simulink library "neuromorphic_blocks"  (R2022a)
settings: Solver=VariableStepAuto  StartTime=0.0  StopTime=10.0  RelTol=1e-3
libraries: $bdroot x31, simulink x7
(part 2 of 2)

== system neuromorphic_blocks/Secondary Blocks ==
  Event Demux : Subsystem  mask(Event Demux){symmetric_box=off, dsyn_signal_pos=0, dsyn_signal_neg=0, dsyn_signal_neg_save=0, gain_signal_pos=1, gain_signal_neg=1, gain_signal_neg_save=1, input=Events, gsyn_pos=0, gsyn_neg=0, gsyn_neg_save=0, dsyn_event_pos=0, dsyn_event_neg=0, dsyn_event_neg_save=0, gain_event_pos=1, gain_event_neg=1, gain_event_neg_save=1}
      mask prompts: symmetric_box "Differentiate positive and negative parameters"; dsyn_signal_pos "Value"; dsyn_signal_neg "Neg"; dsyn_signal_neg_save "Save"; gain_signal_pos "Value"; gain_signal_neg "Neg"; gain_signal_neg_save "Save"; gsyn_pos "Value"; gsyn_neg "Neg"; gsyn_neg_save "Save"; dsyn_event_pos "Value"; dsyn_event_neg "Neg"; dsyn_event_neg_save "Save"; gain_event_pos "Value"; gain_event_neg "Neg"; gain_event_neg_save "Save"
      mask init:
      | mask  = Simulink.Mask.get(gcb);
      |     switch mask.getParameter('input').Value
      |         case 'Events'
      |             %set_param([gcb '/VSNK_ev' ],'LabelModeActiveChoice', 'Events');
      |             %set_param([gcb '/VSNK_s' ],'LabelModeActiveChoice', 'Events');
      |             %set_param([gcb '/VSRC' ],'LabelModeActiveChoice', 'Events');
      |             set_param([gcb '/VSub' ],'LabelModeActiveChoice', 'Events');
      |             %mask.getPortConstraint('inout_main_type').Rule.DataType = {'boolean'};
      |             try
      |                 set_param([gcb '/V'], 'Name', 'Ev');
      |                 set_param([gcb '/V+'], 'Name', 'Ev+');
      |                 set_param([gcb '/V-'], 'Name', 'Ev-');
      |             catch E
      |             end
      |         case 'Voltage'
      |             %set_param([gcb '/VSNK_ev' ],'LabelModeActiveChoice', 'Voltage');
      |             %set_param([gcb '/VSNK_s' ],'LabelModeActiveChoice', 'Voltage');
      |             %set_param([gcb '/VSRC' ],'LabelModeActiveChoice', 'Voltage');
      |             set_param([gcb '/VSub' ],'LabelModeActiveChoice', 'Voltage');
      |             %mask.getPortConstraint('inout_main_type').Rule.DataType = {'double'; 'single'; 'int8'; 'uint8'; 'int16'; 'uint16'; 'int32'; 'uint32'};
      |             try
      |                 set_param([gcb '/Ev'], 'Name', 'V');
      |                 set_param([gcb '/Ev+'], 'Name', 'V+');
      |                 set_param([gcb '/Ev-'], 'Name', 'V-');
      |             catch E
      |             end
      |     end
      | 
      |     suffix_list = {'gsyn', 'dsyn_event', 'gain_event', 'dsyn_signal', 'gain_signal'};
      |     switch mask.getParameter('symmetric_box').Value
      |         case 'off'
      |             for suffix_cell = suffix_list
      |                 suffix = suffix_cell{1};
      |                 mask.getParameter([suffix '_neg']).Value = mask.getParameter([suffix '_pos']).Value;
      |             end
      |         case 'on'
      |             for suffix_cell = suffix_list
      |                 suffix = suffix_cell{1};
      |                 mask.getParameter([suffix '_neg']).Value = mask.getParameter([suffix '_neg_save']).Value;
      |             end
      |     end
      mask Callback symmetric_box:
      | mask  = Simulink.Mask.get(gcb);
      |     switch mask.getParameter('input').Value
      |         case 'Events'
      |             suffix_list = {'dsyn_signal', 'gain_signal'};
      |         case 'Voltage'
      |             suffix_list = {'dsyn_signal', 'gain_signal', 'gsyn', 'dsyn_event', 'gain_event'};
      |     end
      | 
      |     switch mask.getParameter('symmetric_box').Value
      |         case 'on'
      |             for suffix_cell = suffix_list
      |                 suffix = suffix_cell{1};
      |                 %mask.getParameter([suffix '_neg']).Hidden = 'off';
      |                 %mask.getParameter([suffix '_neg_save']).ReadOnly = 'off';
      |                 mask.getParameter([suffix '_neg']).Value = mask.getParameter([suffix '_neg_save']).Value;
      |                 %mask.getParameter([suffix '_neg']).Enabled = 'on';
      |                 mask.getParameter([suffix '_neg']).Visible = 'on';
      |                 mask.getParameter([suffix '_pos']).Prompt = 'Pos';
      |             end
      |         case 'off'
      |             for suffix_cell = suffix_list
      |                 suffix = suffix_cell{1};
      |                 %mask.getParameter([suffix '_neg_save']).Value = mask.getParameter([suffix '_neg']).Value;
      |                 %mask.getParameter([suffix '_neg_save']).ReadOnly = 'on';
      |                 %mask.getParameter([suffix '_neg']).Enabled = 'off';
      |                 mask.getParameter([suffix '_neg']).Visible = 'off';
      |                 mask.getParameter([suffix '_pos']).Prompt = 'Value';
      |                 %mask.getParameter([suffix '_neg']).Value = mask.getParameter([suffix '_pos']).Value;
      |                 %mask.getParameter([suffix '_neg']).Hidden = 'on';
      |             end
      |     end
      mask Callback dsyn_signal_neg:
      | suffix = 'dsyn_signal';
      |     mask  = Simulink.Mask.get(gcb);
      |     switch mask.getParameter('symmetric_box').Value
      |         case 'on'
      |              mask.getParameter([suffix '_neg_save']).Value = mask.getParameter([suffix '_neg']).Value;
      |     end
      mask Callback gain_signal_neg:
      | suffix = 'gain_signal';
      |     mask  = Simulink.Mask.get(gcb);
      |     switch mask.getParameter('symmetric_box').Value
      |         case 'on'
      |              mask.getParameter([suffix '_neg_save']).Value = mask.getParameter([suffix '_neg']).Value;
      |     end
      mask TypeOptions input: Events | Voltage
      mask Callback input:
      | mask = Simulink.Mask.get(gcb);
      |     suffix_list = {'gsyn', 'dsyn_event', 'gain_event'};
      |     switch mask.getParameter('input').Value
      |         case 'Events'
      |             for suffix_cell = suffix_list
      |                 suffix = suffix_cell{1};
      |                 %mask.getParameter([suffix '_pos']).Enabled = 'off';
      |                 mask.getParameter([suffix '_pos']).Visible = 'off';
      |                 %mask.getParameter([suffix '_neg']).Enabled = 'off';
      |                 mask.getParameter([suffix '_neg']).Visible = 'off';
      |                 %mask.getDialogControl([suffix '_text']).Enabled = 'off';
      |                 mask.getDialogControl([suffix '_text']).Visible = 'off';
      |             end
      |         case 'Voltage'
      |             switch mask.getParameter('symmetric_box').Value
      |                 case 'on'
      |                     enable_neg = true;
      |                 case 'off'
      |                     enable_neg = false;
      |             end
      |             for suffix_cell = suffix_list
      |                 suffix = suffix_cell{1};
      |                 %mask.getParameter([suffix '_pos']).Enabled = 'on';
      |                 mask.getParameter([suffix '_pos']).Visible = 'on';
      |                 %mask.getDialogControl([suffix '_text']).Enabled = 'on';
      |                 mask.getDialogControl([suffix '_text']).Visible = 'on';
      |                 if enable_neg
      |                     %mask.getParameter([suffix '_neg']).Enabled = 'on';
      |                     mask.getParameter([suffix '_neg']).Visible = 'on';
      |                 end
      |             end
      |     end
      mask Callback gsyn_neg:
      | suffix = 'gsyn';
      |     mask  = Simulink.Mask.get(gcb);
      |     switch mask.getParameter('symmetric_box').Value
      |         case 'on'
      |              mask.getParameter([suffix '_neg_save']).Value = mask.getParameter([suffix '_neg']).Value;
      |     end
      mask Callback dsyn_event_neg:
      | suffix = 'dsyn_event';
      |     mask  = Simulink.Mask.get(gcb);
      |     switch mask.getParameter('symmetric_box').Value
      |         case 'on'
      |              mask.getParameter([suffix '_neg_save']).Value = mask.getParameter([suffix '_neg']).Value;
      |     end
      mask Callback gain_event_neg:
      | suffix = 'gain_event';
      |     mask  = Simulink.Mask.get(gcb);
      |     switch mask.getParameter('symmetric_box').Value
      |         case 'on'
      |              mask.getParameter([suffix '_neg_save']).Value = mask.getParameter([suffix '_neg']).Value;
      |     end
      mask DialogControl dsyn_signal_text Prompt: Signal Bias
      mask DialogControl gain_signal_text Prompt: Signal Slope
      mask DialogControl input_text Prompt: Input-Output Type
      mask DialogControl gsyn_text Prompt: Event Gain
      mask DialogControl dsyn_event_text Prompt: Event Bias
      mask DialogControl gain_event_text Prompt: Event Slope
      mask Display:
      | simBlockH = get_param(gcb, 'Handle');
      | 
      | 
      | portH = find_system(simBlockH, 'LookUnderMasks', 'on', 'FollowLinks', 'on', 'SearchDepth', 1, 'BlockType', 'Inport');
      | portNames = cellstr(get_param(portH, 'Name'));
      | portNum = cellstr(get_param(portH, 'Port'));
      | for i = 1:length(portNames)
      |     if ~isempty(portNames{i})
      |         num = str2num(['uint8(' portNum{i} ')']);
      |         port_label('input', num, portNames{i});
      |     end
      | end
      | 
      | portH = find_system(simBlockH, 'LookUnderMasks', 'on', 'FollowLinks', 'on', 'SearchDepth', 1, 'BlockType', 'Outport');
      | portNames = cellstr(get_param(portH, 'Name'));
      | portNum = cellstr(get_param(portH, 'Port'));
      | for i = 1:length(portNames)
      |     if ~isempty(portNames{i})
      |         num = str2num(['uint8(' portNum{i} ')']);
      |         port_label('output', num, portNames{i});
      |     end
      | end
  Event Mux : Subsystem  mask(Event Mux){symmetric_box=off, dsyn_signal_pos=0, dsyn_signal_neg=0, dsyn_signal_neg_save=0, gain_signal_pos=1, gain_signal_neg=1, gain_signal_neg_save=1, input=Events, gsyn_pos=0, gsyn_neg=0, gsyn_neg_save=0, dsyn_event_pos=0, dsyn_event_neg=0, dsyn_event_neg_save=0, gain_event_pos=1, gain_event_neg=1, gain_event_neg_save=1}
      mask prompts: symmetric_box "Differentiate positive and negative parameters"; dsyn_signal_pos "Value"; dsyn_signal_neg "Neg"; dsyn_signal_neg_save "Save"; gain_signal_pos "Value"; gain_signal_neg "Neg"; gain_signal_neg_save "Save"; gsyn_pos "Value"; gsyn_neg "Neg"; gsyn_neg_save "Save"; dsyn_event_pos "Value"; dsyn_event_neg "Neg"; dsyn_event_neg_save "Save"; gain_event_pos "Value"; gain_event_neg "Neg"; gain_event_neg_save "Save"
      mask init: same as neuromorphic_blocks/Secondary Blocks/Event Demux
      mask Callback symmetric_box:
      | mask  = Simulink.Mask.get(gcb);
      |     switch mask.getParameter('input').Value
      |         case 'Events'
      |             suffix_list = {'dsyn_signal', 'gain_signal'};
      |         case 'Voltage'
      |             suffix_list = {'dsyn_signal', 'gain_signal', 'gsyn', 'dsyn_event', 'gain_event'};
      |     end
      | 
      |     switch mask.getParameter('symmetric_box').Value
      |         case 'on'
      |             for suffix_cell = suffix_list
      |                 suffix = suffix_cell{1};
      |                 %mask.getParameter([suffix '_neg']).Hidden = 'off';
      |                 %mask.getParameter([suffix '_neg_save']).ReadOnly = 'off';
      |                 mask.getParameter([suffix '_neg']).Value = mask.getParameter([suffix '_neg_save']).Value;
      |                 %mask.getParameter([suffix '_neg']).Enabled = 'on';
      |                 mask.getParameter([suffix '_neg']).Visible = 'on';
      |                 mask.getParameter([suffix '_pos']).Prompt = 'Pos';
      |             end
      |         case 'off'
      |             for suffix_cell = suffix_list
      |                 suffix = suffix_cell{1};
      |                 %mask.getParameter([suffix '_neg_save']).Value = mask.getParameter([suffix '_neg']).Value;
      |                 %mask.getParameter([suffix '_neg_save']).ReadOnly = 'on';
      |                 %mask.getParameter([suffix '_neg']).Enabled = 'off';
      |                 mask.getParameter([suffix '_neg']).Visible = 'off';
      |                 mask.getParameter([suffix '_pos']).Prompt = 'Value';
      |                 %mask.getParameter([suffix '_neg']).Value = mask.getParameter([suffix '_pos']).Value;
      |                 %mask.getParameter([suffix '_neg']).Hidden = 'on';
      |             end
      |     end
      mask Callback dsyn_signal_neg:
      | suffix = 'dsyn_signal';
      |     mask  = Simulink.Mask.get(gcb);
      |     switch mask.getParameter('symmetric_box').Value
      |         case 'on'
      |              mask.getParameter([suffix '_neg_save']).Value = mask.getParameter([suffix '_neg']).Value;
      |     end
      mask Callback gain_signal_neg:
      | suffix = 'gain_signal';
      |     mask  = Simulink.Mask.get(gcb);
      |     switch mask.getParameter('symmetric_box').Value
      |         case 'on'
      |              mask.getParameter([suffix '_neg_save']).Value = mask.getParameter([suffix '_neg']).Value;
      |     end
      mask TypeOptions input: Events | Voltage
      mask Callback input:
      | mask = Simulink.Mask.get(gcb);
      |     suffix_list = {'gsyn', 'dsyn_event', 'gain_event'};
      |     switch mask.getParameter('input').Value
      |         case 'Events'
      |             for suffix_cell = suffix_list
      |                 suffix = suffix_cell{1};
      |                 %mask.getParameter([suffix '_pos']).Enabled = 'off';
      |                 mask.getParameter([suffix '_pos']).Visible = 'off';
      |                 %mask.getParameter([suffix '_neg']).Enabled = 'off';
      |                 mask.getParameter([suffix '_neg']).Visible = 'off';
      |                 %mask.getDialogControl([suffix '_text']).Enabled = 'off';
      |                 mask.getDialogControl([suffix '_text']).Visible = 'off';
      |             end
      |         case 'Voltage'
      |             switch mask.getParameter('symmetric_box').Value
      |                 case 'on'
      |                     enable_neg = true;
      |                 case 'off'
      |                     enable_neg = false;
      |             end
      |             for suffix_cell = suffix_list
      |                 suffix = suffix_cell{1};
      |                 %mask.getParameter([suffix '_pos']).Enabled = 'on';
      |                 mask.getParameter([suffix '_pos']).Visible = 'on';
      |                 %mask.getDialogControl([suffix '_text']).Enabled = 'on';
      |                 mask.getDialogControl([suffix '_text']).Visible = 'on';
      |                 if enable_neg
      |                     %mask.getParameter([suffix '_neg']).Enabled = 'on';
      |                     mask.getParameter([suffix '_neg']).Visible = 'on';
      |                 end
      |             end
      |     end
      mask Callback gsyn_neg:
      | suffix = 'gsyn';
      |     mask  = Simulink.Mask.get(gcb);
      |     switch mask.getParameter('symmetric_box').Value
      |         case 'on'
      |              mask.getParameter([suffix '_neg_save']).Value = mask.getParameter([suffix '_neg']).Value;
      |     end
      mask Callback dsyn_event_neg:
      | suffix = 'dsyn_event';
      |     mask  = Simulink.Mask.get(gcb);
      |     switch mask.getParameter('symmetric_box').Value
      |         case 'on'
      |              mask.getParameter([suffix '_neg_save']).Value = mask.getParameter([suffix '_neg']).Value;
      |     end
      mask Callback gain_event_neg:
      | suffix = 'gain_event';
      |     mask  = Simulink.Mask.get(gcb);
      |     switch mask.getParameter('symmetric_box').Value
      |         case 'on'
      |              mask.getParameter([suffix '_neg_save']).Value = mask.getParameter([suffix '_neg']).Value;
      |     end
      mask DialogControl dsyn_signal_text Prompt: Signal Bias
      mask DialogControl gain_signal_text Prompt: Signal Slope
      mask DialogControl input_text Prompt: Input-Output Type
      mask DialogControl gsyn_text Prompt: Event Gain
      mask DialogControl dsyn_event_text Prompt: Event Bias
      mask DialogControl gain_event_text Prompt: Event Slope
      mask Display:
      | simBlockH = get_param(gcb, 'Handle');
      | 
      | 
      | portH = find_system(simBlockH, 'LookUnderMasks', 'on', 'FollowLinks', 'on', 'SearchDepth', 1, 'BlockType', 'Inport');
      | portNames = cellstr(get_param(portH, 'Name'));
      | portNum = cellstr(get_param(portH, 'Port'));
      | for i = 1:length(portNames)
      |     if ~isempty(portNames{i})
      |         num = str2num(['uint8(' portNum{i} ')']);
      |         port_label('input', num, portNames{i});
      |     end
      | end
      | 
      | portH = find_system(simBlockH, 'LookUnderMasks', 'on', 'FollowLinks', 'on', 'SearchDepth', 1, 'BlockType', 'Outport');
      | portNames = cellstr(get_param(portH, 'Name'));
      | portNum = cellstr(get_param(portH, 'Port'));
      | for i = 1:length(portNames)
      |     if ~isempty(portNames{i})
      |         num = str2num(['uint8(' portNum{i} ')']);
      |         port_label('output', num, portNames{i});
      |     end
      | end
  Noise on Signal : Subsystem  mask(Noise on Signal){noise_pwr=0, timescale=0.004, rel_timescale=1, seed=-1, seed_mem=randi([0, 100000])}
      mask prompts: noise_pwr "Value"; timescale "Value"; rel_timescale "Value"; seed "Value"
      mask init: same as neuromorphic_blocks/Events Transmission Blocks/Event Loss
      mask DialogControl noise_pwr_text Prompt: Noise Power
      mask DialogControl timescale_text Prompt: Timescale
      mask DialogControl rel_timescale_text Prompt: Relative Timescale
      mask DialogControl seed_text Prompt: Seed (-1 for random seed)
      mask Display:
      | xscale = 0.8;
      | yscale = 0.8;
      | 
      | r = [-0.4326
      |    -1.6656
      |     0.1253
      |     0.2877
      |    -1.1465
      |     1.1909
      |     1.1892
      |    -0.0376
      |     0.3273
      |     0.1746
      |    -0.1867
      |     0.7258]';
      | 
      | r2 = repelem(r,2);
      | r3 = r2 - min(r2);
      | r4 = r3/max(r3);
      | r5 = r4*yscale + (1-yscale)/2;
      | 
      | 
      | t = [1 repelem(2:12,2) 13];
      | t2 = t - min(t);
      | t3 = t2/max(t2);
      | t4 = t3*xscale + (1-xscale)/2;
      | 
      | 
      | plot(t4, r5);

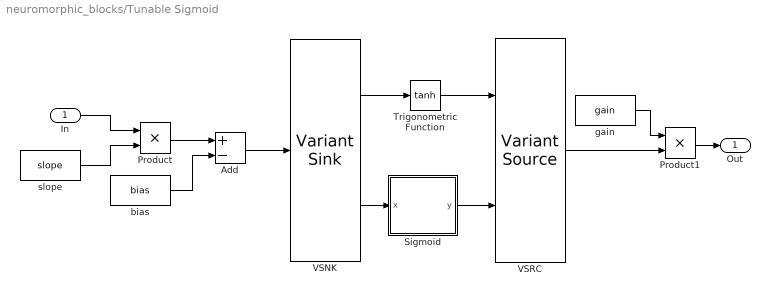
== system neuromorphic_blocks/Tunable Sigmoid ==
  In : Inport
  Add : Sum  Inputs=+-
  Product : Product
  Product1 : Product
  Sigmoid : Subsystem
  Trigonometric Function : Trigonometry  Operator=tanh
  VSNK : VariantSink  VariantControlMode=label  LabelModeActiveChoice=Sigmoid  ShowConditionOnBlock=on
  VSRC : VariantSource  VariantControlMode=label  LabelModeActiveChoice=Sigmoid  ShowConditionOnBlock=on
  bias : Constant  Value=bias
  gain : Constant  Value=gain
  slope : Constant  Value=slope
  Out : Outport
  wires:
  VSNK/1 -> Trigonometric Function/1
  slope/1 -> Product/2
  In/1 -> Product/1
  Add/1 -> VSNK/1
  Product/1 -> Add/1
  bias/1 -> Add/2
  VSRC/1 -> Product1/2
  Product1/1 -> Out/1
  gain/1 -> Product1/1
  VSNK/2 -> Sigmoid/1(x)
  Sigmoid/1(y) -> VSRC/2
  Trigonometric Function/1 -> VSRC/1

== system neuromorphic_blocks/Events Transmission Blocks/Continuous to Event ==
  In : Inport
  Constant2 : Constant  Value=thresh
  Relational Operator : RelationalOperator  OutDataTypeStr=boolean  RndMeth=Simplest  InputSameDT=off
  Out : Outport  OutDataTypeStr=boolean
  wires:
  Constant2/1 -> Relational Operator/2
  In/1 -> Relational Operator/1
  Relational Operator/1 -> Out/1

== system neuromorphic_blocks/Events Transmission Blocks/Event Loss ==
  In : Inport
  Constant4 : Constant  Value=0  OutDataTypeStr=Inherit: Inherit via back propagation
  Generate Random Number on Positive : Subsystem  TreatAsAtomicUnit=on
  Pipe Signal : Switch  Threshold=loss_prob  SaturateOnIntegerOverflow=off  InputSameDT=off
  Out : Outport
  wires:
  Generate Random Number on Positive/1(Out1) -> Pipe Signal/2
  In/1 -> Pipe Signal/1, Generate Random Number on Positive/Trigger
  Constant4/1 -> Pipe Signal/3
  Pipe Signal/1 -> Out/1

== system neuromorphic_blocks/Events Transmission Blocks/Event to Continuous ==
  In : Inport  OutDataTypeStr=boolean
  Gain : Gain  Gain=gain  OutDataTypeStr=double
  Out : Outport  OutDataTypeStr=double
  wires:
  In/1 -> Gain/1
  Gain/1 -> Out/1

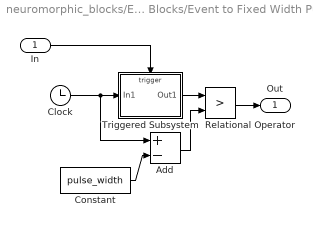
== system neuromorphic_blocks/Events Transmission Blocks/Event to Fixed Width Pulse ==
  In : Inport
  Add : Sum  Inputs=+-
  Clock : Clock
  Constant : Constant  Value=pulse_width
  Relational Operator : RelationalOperator  Operator=>  OutDataTypeStr=boolean  RndMeth=Simplest  InputSameDT=off
  Triggered Subsystem : Subsystem  TreatAsAtomicUnit=on
  Out : Outport
  wires:
  Constant/1 -> Add/2
  Triggered Subsystem/1(Out1) -> Relational Operator/1
  Add/1 -> Relational Operator/2
  Clock/1 -> Add/1, Triggered Subsystem/1(In1)
  Relational Operator/1 -> Out/1
  In/1 -> Triggered Subsystem/Trigger

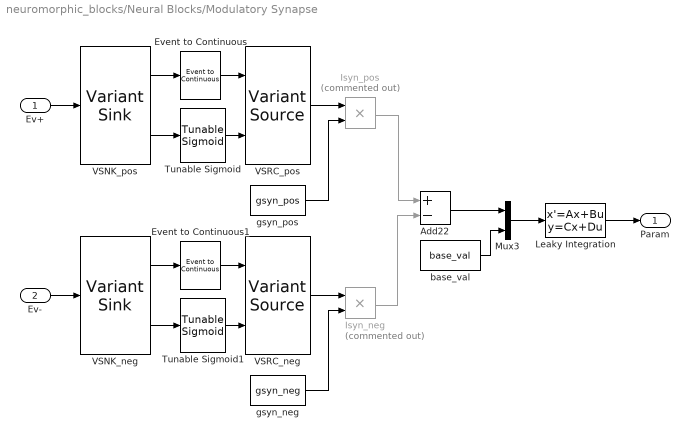
== system neuromorphic_blocks/Neural Blocks/Modulatory Synapse ==
  Ev+ : Inport
  Ev- : Inport  Port=2
  Add22 : Sum  Inputs=+-
  Event to Continuous : $bdroot/Events Transmission Blocks/Event to Continuous  gain=1
  Event to Continuous1 : $bdroot/Events Transmission Blocks/Event to Continuous  gain=1
  Isyn_neg : Product  Commented=on
  Isyn_pos : Product  Commented=on
  Leaky Integration : StateSpace  A=-1/(timescale*rel_timescale)  B=[1 1/(timescale*rel_timescale)]  D=[0 0]  InitialCondition=base_val  ParameterTunability=Unconstrained
  Mux3 : Mux  Inputs=2
  Tunable Sigmoid : $bdroot/Tunable Sigmoid  nonlinearity_type=Sigmoid  gain_source=Internal  gain=1  bias=dsyn_pos  slope=msyn_pos
  Tunable Sigmoid1 : $bdroot/Tunable Sigmoid  nonlinearity_type=Sigmoid  gain_source=Internal  gain=1  bias=dsyn_neg  slope=msyn_neg
  VSNK_neg : VariantSink  VariantControlMode=label  LabelModeActiveChoice=Events  ShowConditionOnBlock=on
  VSNK_pos : VariantSink  VariantControlMode=label  LabelModeActiveChoice=Events  ShowConditionOnBlock=on
  VSRC_neg : VariantSource  VariantControlMode=label  LabelModeActiveChoice=Events  ShowConditionOnBlock=on
  VSRC_pos : VariantSource  VariantControlMode=label  LabelModeActiveChoice=Events  ShowConditionOnBlock=on
  base_val : Constant  Value=base_val
  gsyn_neg : Constant  Value=gsyn_neg
  gsyn_pos : Constant  Value=gsyn_pos
  Param : Outport
  wires:
  base_val/1 -> Mux3/2
  Mux3/1 -> Leaky Integration/1
  Leaky Integration/1 -> Param/1
  Ev+/1 -> VSNK_pos/1
  Add22/1 -> Mux3/1
  Isyn_pos/1 -> Add22/1
  Isyn_neg/1 -> Add22/2
  VSNK_pos/1 -> Event to Continuous/1
  Event to Continuous/1 -> VSRC_pos/1
  Tunable Sigmoid/1 -> VSRC_pos/2
  VSNK_pos/2 -> Tunable Sigmoid/1
  VSRC_pos/1 -> Isyn_pos/1
  gsyn_pos/1 -> Isyn_pos/2
  VSRC_neg/1 -> Isyn_neg/1
  gsyn_neg/1 -> Isyn_neg/2
  Event to Continuous1/1 -> VSRC_neg/1
  VSNK_neg/2 -> Tunable Sigmoid1/1
  VSNK_neg/1 -> Event to Continuous1/1
  Tunable Sigmoid1/1 -> VSRC_neg/2
  Ev-/1 -> VSNK_neg/1

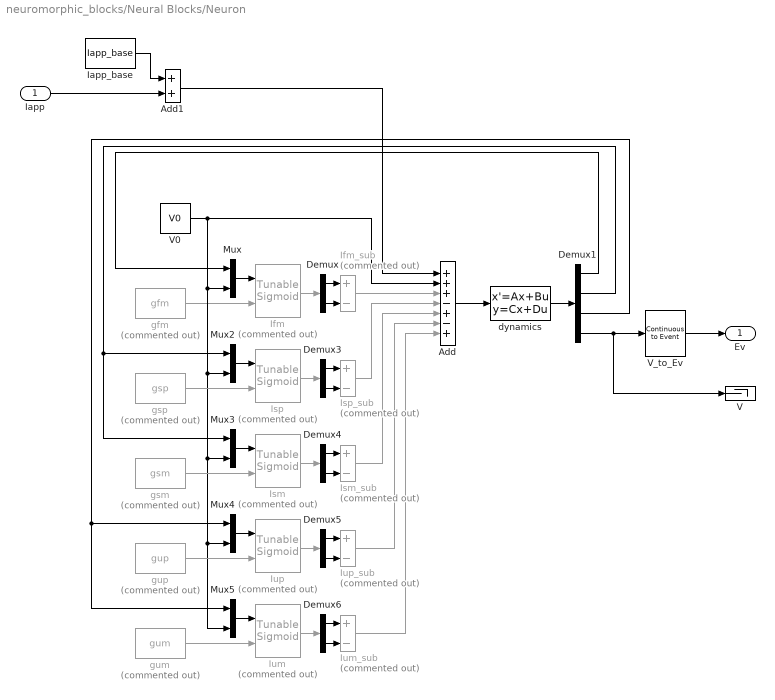
== system neuromorphic_blocks/Neural Blocks/Neuron ==
  Iapp : Inport
  Add : Sum  Inputs=+++-+-+
  Add1 : Sum
  Demux{,3..6} (5 alike) : Demux  Outputs=2
  Demux1 : Demux
  Iapp_base : Constant  Value=Iapp_base
  Ifm : $bdroot/Tunable Sigmoid  Commented=on  nonlinearity_type=Tanh  gain_source=External  gain=0  bias=dfm  slope=mfm
  Ifm_sub : Sum  Commented=on  Inputs=+-
  Ism : $bdroot/Tunable Sigmoid  Commented=on  nonlinearity_type=Tanh  gain_source=External  gain=0  bias=dsm  slope=msm
  Ism_sub : Sum  Commented=on  Inputs=+-
  Isp : $bdroot/Tunable Sigmoid  Commented=on  nonlinearity_type=Tanh  gain_source=External  gain=0  bias=dsp  slope=msp
  Isp_sub : Sum  Commented=on  Inputs=+-
  Ium : $bdroot/Tunable Sigmoid  Commented=on  nonlinearity_type=Tanh  gain_source=External  gain=0  bias=dum  slope=mum
  Ium_sub : Sum  Commented=on  Inputs=+-
  Iup : $bdroot/Tunable Sigmoid  Commented=on  nonlinearity_type=Tanh  gain_source=External  gain=0  bias=dup  slope=mup
  Iup_sub : Sum  Commented=on  Inputs=+-
  Mux{,2..5} (5 alike) : Mux  Inputs=2
  V : Terminator
  V0 : Constant  Value=V0
  V_to_Ev : $bdroot/Events Transmission Blocks/Continuous to Event  thresh=tresh
  dynamics : StateSpace  A=[-1/rel_fast 0 0 1/rel_fast; 0 -1/rel_slow 0 1/rel_slow; 0 0 -1/rel_ultraslow 1/rel_ultraslow; 0 0 0 -1/rel_membrane]/(timescale)  B=[0; 0; 0; 1/rel_membrane]/timescale  C=[1 0 0 0; 0 1 0 0; 0 0 1 0; 0 0 0 1]  D=[0; 0; 0; 0]  InitialCondition=[V0; V0; V0; V0]
  gfm : Constant  Commented=on  Value=gfm
  gsm : Constant  Commented=on  Value=gsm
  gsp : Constant  Commented=on  Value=gsp
  gum : Constant  Commented=on  Value=gum
  gup : Constant  Commented=on  Value=gup
  Ev : Outport
  wires:
  dynamics/1 -> Demux1/1
  Add1/1 -> Add/1
  gfm/1 -> Ifm/2
  Iapp_base/1 -> Add1/1
  Demux1/1 -> Mux/1
  Add/1 -> dynamics/1
  V0/1 -> Mux/2, Mux2/2, Mux5/2, Mux4/2, Mux3/2, Add/2
  Iapp/1 -> Add1/2
  Demux1/3 -> Mux4/1, Mux5/1
  Demux1/4 -> V/1, V_to_Ev/1
  Demux1/2 -> Mux3/1, Mux2/1
  V_to_Ev/1 -> Ev/1
  Mux/1 -> Ifm/1
  Ifm/1 -> Demux/1
  Demux/1 -> Ifm_sub/1
  Demux/2 -> Ifm_sub/2
  Ifm_sub/1 -> Add/3
  Demux3/1 -> Isp_sub/1
  Demux3/2 -> Isp_sub/2
  Mux2/1 -> Isp/1
  Isp/1 -> Demux3/1
  gsp/1 -> Isp/2
  Isp_sub/1 -> Add/4
  Demux4/1 -> Ism_sub/1
  Demux4/2 -> Ism_sub/2
  Mux3/1 -> Ism/1
  Ism/1 -> Demux4/1
  gsm/1 -> Ism/2
  Demux5/1 -> Iup_sub/1
  Demux5/2 -> Iup_sub/2
  Mux4/1 -> Iup/1
  Iup/1 -> Demux5/1
  gup/1 -> Iup/2
  Ism_sub/1 -> Add/5
  Iup_sub/1 -> Add/6
  Ium/1 -> Demux6/1
  Mux5/1 -> Ium/1
  gum/1 -> Ium/2
  Demux6/2 -> Ium_sub/2
  Demux6/1 -> Ium_sub/1
  Ium_sub/1 -> Add/7

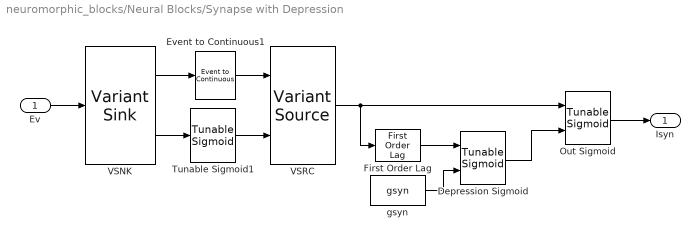
== system neuromorphic_blocks/Neural Blocks/Synapse with Depression ==
  Ev : Inport
  Depression Sigmoid : $bdroot/Tunable Sigmoid  nonlinearity_type=Sigmoid  gain_source=External  gain=0  bias=dsyn_dep  slope=-msyn_dep
  Event to Continuous1 : $bdroot/Events Transmission Blocks/Event to Continuous  gain=1
  First Order Lag : $bdroot/First Order Lag  gain=1  timescale=timescale  rel_timescale=rel_timescale
  Out Sigmoid : $bdroot/Tunable Sigmoid  nonlinearity_type=Sigmoid  gain_source=External  gain=0  bias=dsyn  slope=msyn
  Tunable Sigmoid1 : $bdroot/Tunable Sigmoid  nonlinearity_type=Sigmoid  gain_source=Internal  gain=gsyn_in  bias=dsyn_in  slope=msyn_in
  VSNK : VariantSink  VariantControlMode=label  LabelModeActiveChoice=Events  ShowConditionOnBlock=on
  VSRC : VariantSource  VariantControlMode=label  LabelModeActiveChoice=Events  ShowConditionOnBlock=on
  gsyn : Constant  Value=gsyn
  Isyn : Outport
  wires:
  VSRC/1 -> First Order Lag/1, Out Sigmoid/1
  Out Sigmoid/1 -> Isyn/1
  gsyn/1 -> Depression Sigmoid/2
  VSNK/1 -> Event to Continuous1/1
  Event to Continuous1/1 -> VSRC/1
  Tunable Sigmoid1/1 -> VSRC/2
  VSNK/2 -> Tunable Sigmoid1/1
  Ev/1 -> VSNK/1
  Depression Sigmoid/1 -> Out Sigmoid/2
  First Order Lag/1 -> Depression Sigmoid/1

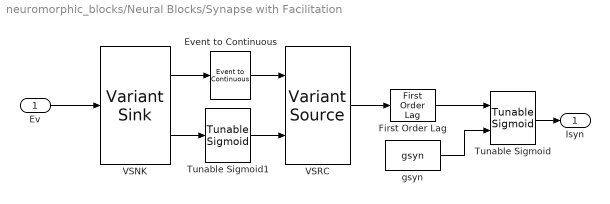
== system neuromorphic_blocks/Neural Blocks/Synapse with Facilitation ==
  Ev : Inport
  Event to Continuous : $bdroot/Events Transmission Blocks/Event to Continuous  gain=1
  First Order Lag : $bdroot/First Order Lag  gain=1  timescale=timescale  rel_timescale=rel_timescale
  Tunable Sigmoid : $bdroot/Tunable Sigmoid  nonlinearity_type=Sigmoid  gain_source=External  gain=0  bias=dsyn  slope=msyn
  Tunable Sigmoid1 : $bdroot/Tunable Sigmoid  nonlinearity_type=Sigmoid  gain_source=Internal  gain=gsyn_in  bias=dsyn_in  slope=msyn_in
  VSNK : VariantSink  VariantControlMode=label  LabelModeActiveChoice=Events  ShowConditionOnBlock=on
  VSRC : VariantSource  VariantControlMode=label  LabelModeActiveChoice=Events  ShowConditionOnBlock=on
  gsyn : Constant  Value=gsyn
  Isyn : Outport
  wires:
  First Order Lag/1 -> Tunable Sigmoid/1
  Tunable Sigmoid/1 -> Isyn/1
  gsyn/1 -> Tunable Sigmoid/2
  Ev/1 -> VSNK/1
  VSNK/2 -> Tunable Sigmoid1/1
  VSNK/1 -> Event to Continuous/1
  Tunable Sigmoid1/1 -> VSRC/2
  Event to Continuous/1 -> VSRC/1
  VSRC/1 -> First Order Lag/1

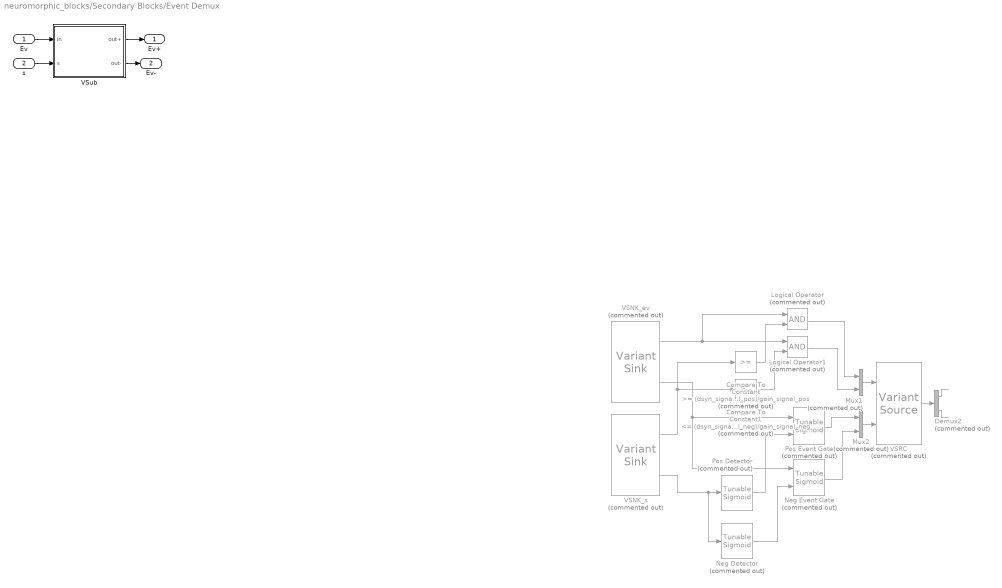
== system neuromorphic_blocks/Secondary Blocks/Event Demux ==
  Ev : Inport
  s : Inport  Port=2
  Compare To Constant : simulink/Logic and Bit Operations/Compare To Constant  Commented=on  relop=>=  const=(dsyn_signal_pos)/gain_signal_pos  OutDataTypeStr=boolean
  Compare To Constant1 : simulink/Logic and Bit Operations/Compare To Constant  Commented=on  relop=<=  const=(dsyn_signal_neg)/gain_signal_neg  OutDataTypeStr=boolean
  Demux2 : Demux  Commented=on  Outputs=2
  Logical Operator : Logic  Commented=on  AllPortsSameDT=off  OutDataTypeStr=boolean
  Logical Operator1 : Logic  Commented=on  AllPortsSameDT=off  OutDataTypeStr=boolean
  Mux1 : Mux  Commented=on  Inputs=2
  Mux2 : Mux  Commented=on  Inputs=2
  Neg Detector : $bdroot/Tunable Sigmoid  Commented=on  nonlinearity_type=Sigmoid  gain_source=Internal  gain=gsyn_neg  bias=-dsyn_signal_neg  slope=-gain_signal_neg
  Neg Event Gate : $bdroot/Tunable Sigmoid  Commented=on  nonlinearity_type=Sigmoid  gain_source=External  gain=0  bias=dsyn_event_neg  slope=gain_event_neg
  Pos Detector : $bdroot/Tunable Sigmoid  Commented=on  nonlinearity_type=Sigmoid  gain_source=Internal  gain=gsyn_pos  bias=dsyn_signal_pos  slope=gain_signal_pos
  Pos Event Gate : $bdroot/Tunable Sigmoid  Commented=on  nonlinearity_type=Sigmoid  gain_source=External  gain=0  bias=dsyn_event_pos  slope=gain_event_pos
  VSNK_ev : VariantSink  Commented=on  VariantControlMode=label  LabelModeActiveChoice=Events  ShowConditionOnBlock=on
  VSNK_s : VariantSink  Commented=on  VariantControlMode=label  LabelModeActiveChoice=Events  ShowConditionOnBlock=on
  VSRC : VariantSource  Commented=on  VariantControlMode=label  LabelModeActiveChoice=Events  ShowConditionOnBlock=on
  VSub : Subsystem  Variant=on  VariantControlMode=label  LabelModeActiveChoice=Events
  Ev+ : Outport
  Ev- : Outport  Port=2
  wires:
  Ev/1 -> VSub/1(in)
  s/1 -> VSub/2(s)
  Logical Operator1/1 -> Mux1/2
  Demux2/2 -> ?
  Mux2/1 -> VSRC/2
  VSNK_ev/2 -> Neg Event Gate/1, Pos Event Gate/1
  VSNK_s/1 -> Compare To Constant/1, Compare To Constant1/1
  Logical Operator/1 -> Mux1/1
  Demux2/1 -> ?
  Neg Detector/1 -> Neg Event Gate/2
  VSRC/1 -> Demux2/1
  VSNK_ev/1 -> Logical Operator1/1, Logical Operator/1
  Neg Event Gate/1 -> Mux2/2
  Mux1/1 -> VSRC/1
  Pos Detector/1 -> Pos Event Gate/2
  VSNK_s/2 -> Neg Detector/1, Pos Detector/1
  Compare To Constant/1 -> Logical Operator/2
  Compare To Constant1/1 -> Logical Operator1/2
  Pos Event Gate/1 -> Mux2/1
  VSub/2(out-) -> Ev-/1
  VSub/1(out+) -> Ev+/1

== system neuromorphic_blocks/Secondary Blocks/Event Mux ==
  Ev+ : Inport
  Ev- : Inport  Port=2
  s : Inport  Port=3
  VSub : Subsystem  Variant=on  VariantControlMode=label  LabelModeActiveChoice=Events
  Ev : Outport
  wires:
  Ev+/1 -> VSub/1(in+)
  Ev-/1 -> VSub/2(in-)
  VSub/1(out) -> Ev/1
  s/1 -> VSub/3(s)

== system neuromorphic_blocks/Secondary Blocks/Noise on Signal ==
  In : Inport
  Add : Sum
  Noise : simulink/Sources/Band-Limited White Noise  Cov=noise_pwr  Ts=timescale*rel_timescale  seed=seed_mem
  Out : Outport
  wires:
  In/1 -> Add/2
  Add/1 -> Out/1
  Noise/1 -> Add/1

== system neuromorphic_blocks/Tunable Sigmoid/Sigmoid ==
  x : Inport
  Constant : Constant
  Gain : Gain  Gain=2
  Gain1 : Gain  Gain=0.5
  Sum : Sum  Inputs=|++
  Trigonometric Function : Trigonometry  Operator=tanh
  y : Outport
  wires:
  Gain/1 -> Trigonometric Function/1
  x/1 -> Gain/1
  Trigonometric Function/1 -> Sum/1
  Constant/1 -> Sum/2
  Sum/1 -> Gain1/1
  Gain1/1 -> y/1

== system neuromorphic_blocks/Events Transmission Blocks/Event Loss/Generate Random Number on Positive ==
  Trigger : TriggerPort  TriggerType=either  VariantControl=(inherit)  ShowOutputPort=on
  Constant : Constant  Value=0
  Switch : Switch  SaturateOnIntegerOverflow=off  InputSameDT=off
  Uniform Random Number1 : UniformRandomNumber  Minimum=0  Seed=seed_mem
  Out1 : Outport
  wires:
  Constant/1 -> Switch/3
  Trigger/1 -> Switch/2
  Uniform Random Number1/1 -> Switch/1
  Switch/1 -> Out1/1

== system neuromorphic_blocks/Events Transmission Blocks/Event to Fixed Width Pulse/Triggered Subsystem ==
  In1 : Inport
  Trigger : TriggerPort  VariantControl=(inherit)  InitialTriggerSignalState=zero
  Out1 : Outport  InitialOutput=-pulse_width
  wires:
  In1/1 -> Out1/1

== system neuromorphic_blocks/Secondary Blocks/Event Demux/VSub ==
  in : Inport
  s : Inport  Port=2
  Events : Subsystem  VariantControl=Events
  Voltage : Subsystem  VariantControl=Voltage
  out+ : Outport
  out- : Outport  Port=2

== system neuromorphic_blocks/Secondary Blocks/Event Mux/VSub ==
  in+ : Inport
  in- : Inport  Port=2
  s : Inport  Port=3
  Events : Subsystem  VariantControl=Events
  Voltage : Subsystem  VariantControl=Voltage
  out : Outport

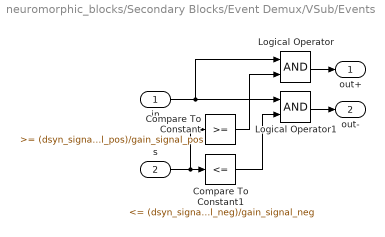
== system neuromorphic_blocks/Secondary Blocks/Event Demux/VSub/Events ==
  in : Inport
  s : Inport  Port=2
  Compare To Constant : simulink/Logic and Bit Operations/Compare To Constant  relop=>=  const=(dsyn_signal_pos)/gain_signal_pos  OutDataTypeStr=boolean
  Compare To Constant1 : simulink/Logic and Bit Operations/Compare To Constant  relop=<=  const=(dsyn_signal_neg)/gain_signal_neg  OutDataTypeStr=boolean
  Logical Operator : Logic  AllPortsSameDT=off  OutDataTypeStr=boolean
  Logical Operator1 : Logic  AllPortsSameDT=off  OutDataTypeStr=boolean
  out+ : Outport
  out- : Outport  Port=2
  wires:
  Compare To Constant/1 -> Logical Operator/2
  Compare To Constant1/1 -> Logical Operator1/2
  in/1 -> Logical Operator/1, Logical Operator1/1
  Logical Operator1/1 -> out-/1
  Logical Operator/1 -> out+/1
  s/1 -> Compare To Constant/1, Compare To Constant1/1

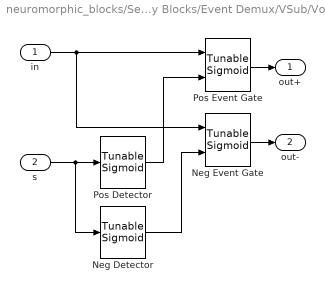
== system neuromorphic_blocks/Secondary Blocks/Event Demux/VSub/Voltage ==
  in : Inport
  s : Inport  Port=2
  Neg Detector : $bdroot/Tunable Sigmoid  nonlinearity_type=Sigmoid  gain_source=Internal  gain=gsyn_neg  bias=-dsyn_signal_neg  slope=-gain_signal_neg
  Neg Event Gate : $bdroot/Tunable Sigmoid  nonlinearity_type=Sigmoid  gain_source=External  gain=0  bias=dsyn_event_neg  slope=gain_event_neg
  Pos Detector : $bdroot/Tunable Sigmoid  nonlinearity_type=Sigmoid  gain_source=Internal  gain=gsyn_pos  bias=dsyn_signal_pos  slope=gain_signal_pos
  Pos Event Gate : $bdroot/Tunable Sigmoid  nonlinearity_type=Sigmoid  gain_source=External  gain=0  bias=dsyn_event_pos  slope=gain_event_pos
  out+ : Outport
  out- : Outport  Port=2
  wires:
  Neg Detector/1 -> Neg Event Gate/2
  in/1 -> Pos Event Gate/1, Neg Event Gate/1
  s/1 -> Neg Detector/1, Pos Detector/1
  Pos Detector/1 -> Pos Event Gate/2
  Pos Event Gate/1 -> out+/1
  Neg Event Gate/1 -> out-/1

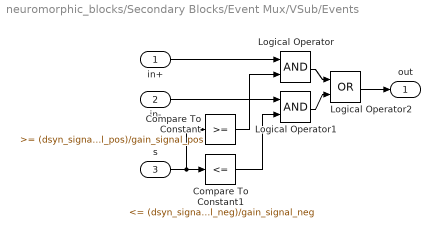
== system neuromorphic_blocks/Secondary Blocks/Event Mux/VSub/Events ==
  in+ : Inport
  in- : Inport  Port=2
  s : Inport  Port=3
  Compare To Constant : simulink/Logic and Bit Operations/Compare To Constant  relop=>=  const=(dsyn_signal_pos)/gain_signal_pos  OutDataTypeStr=boolean
  Compare To Constant1 : simulink/Logic and Bit Operations/Compare To Constant  relop=<=  const=(dsyn_signal_neg)/gain_signal_neg  OutDataTypeStr=boolean
  Logical Operator : Logic  AllPortsSameDT=off  OutDataTypeStr=boolean
  Logical Operator1 : Logic  AllPortsSameDT=off  OutDataTypeStr=boolean
  Logical Operator2 : Logic  Operator=OR  AllPortsSameDT=off  OutDataTypeStr=boolean
  out : Outport
  wires:
  Compare To Constant/1 -> Logical Operator/2
  Compare To Constant1/1 -> Logical Operator1/2
  in+/1 -> Logical Operator/1
  in-/1 -> Logical Operator1/1
  s/1 -> Compare To Constant/1, Compare To Constant1/1
  Logical Operator2/1 -> out/1
  Logical Operator1/1 -> Logical Operator2/2
  Logical Operator/1 -> Logical Operator2/1

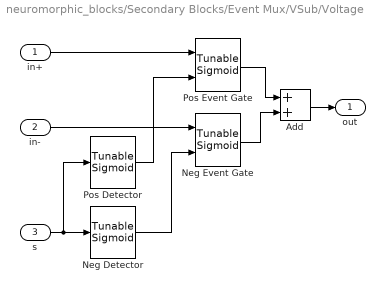
== system neuromorphic_blocks/Secondary Blocks/Event Mux/VSub/Voltage ==
  in+ : Inport
  in- : Inport  Port=2
  s : Inport  Port=3
  Add : Sum
  Neg Detector : $bdroot/Tunable Sigmoid  nonlinearity_type=Sigmoid  gain_source=Internal  gain=gsyn_neg  bias=-dsyn_signal_neg  slope=-gain_signal_neg
  Neg Event Gate : $bdroot/Tunable Sigmoid  nonlinearity_type=Sigmoid  gain_source=External  gain=0  bias=dsyn_event_neg  slope=gain_event_neg
  Pos Detector : $bdroot/Tunable Sigmoid  nonlinearity_type=Sigmoid  gain_source=Internal  gain=gsyn_pos  bias=dsyn_signal_pos  slope=gain_signal_pos
  Pos Event Gate : $bdroot/Tunable Sigmoid  nonlinearity_type=Sigmoid  gain_source=External  gain=0  bias=dsyn_event_pos  slope=gain_event_pos
  out : Outport
  wires:
  Add/1 -> out/1
  Neg Event Gate/1 -> Add/2
  Pos Detector/1 -> Pos Event Gate/2
  in+/1 -> Pos Event Gate/1
  in-/1 -> Neg Event Gate/1
  Pos Event Gate/1 -> Add/1
  Neg Detector/1 -> Neg Event Gate/2
  s/1 -> Neg Detector/1, Pos Detector/1
